simulink model "EXP1_EX13"  (R2021b)
settings: Solver=VariableStepAuto  StartTime=0.0  StopTime=20.0  RelTol=1e-3
values from neighbouring files (symbols this model uses):
  kp = eye(2)    [EXP1.m]
  u1 = 0    [EXP1.m]
  u2 = 1    [EXP1.m]
settings Model: Creator=luang  LastModifiedBy=luang

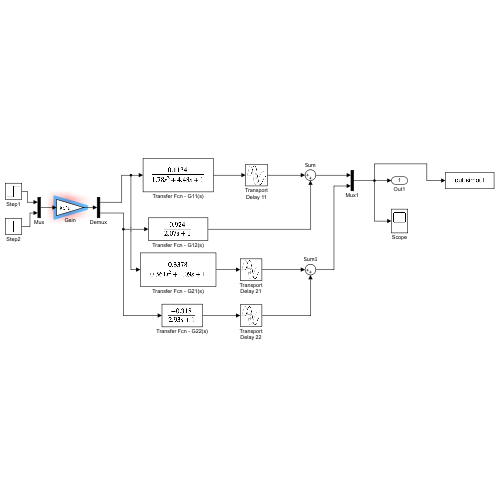
[thumbnail: Simulink's stored preview of the top-level diagram]
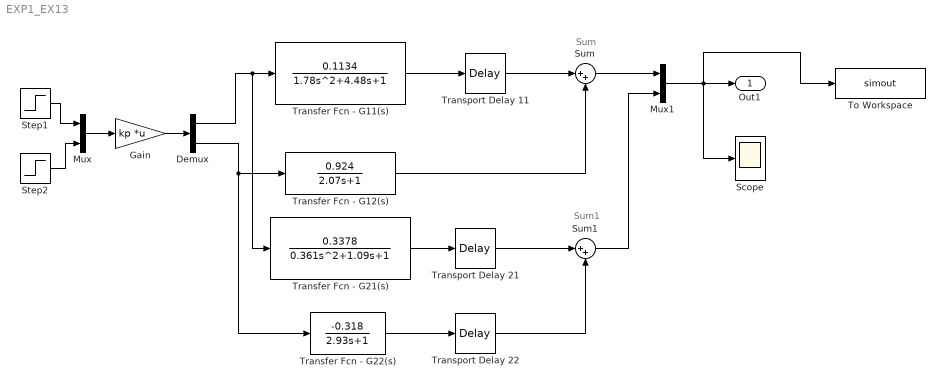
== system EXP1_EX13 ==
  note: Sum
  note: Sum1
  Demux : Demux  Outputs=2
  Gain : Gain  Gain=kp  Multiplication=Matrix(K*u)
  Mux : Mux  Inputs=2
  Mux1 : Mux  Inputs=2
  Scope : Scope
  Step1 : Step  After=u1  SampleTime=0
  Step2 : Step  After=u2  SampleTime=0
  Sum : Sum  Inputs=|++
  Sum1 : Sum  Inputs=|++
  To Workspace : ToWorkspace  VariableName=simout  SaveFormat=Structure With Time  SampleTime=-1
  Transfer Fcn - G11(s) : TransferFcn  Numerator=[0.1134]  Denominator=[1.78 4.48 1]  ContinuousStateAttributes='G11'
  Transfer Fcn - G12(s) : TransferFcn  Numerator=[0.924]  Denominator=[2.07 1]
  Transfer Fcn - G21(s) : TransferFcn  Numerator=[0.3378]  Denominator=[0.361 1.09 1]
  Transfer Fcn - G22(s) : TransferFcn  Numerator=[-0.318]  Denominator=[2.93 1]
  Transport Delay 11 : TransportDelay  DelayTime=0.72
  Transport Delay 21 : TransportDelay  DelayTime=0.3
  Transport Delay 22 : TransportDelay  DelayTime=1.29
  Out1 : Outport
  wires:
  Demux/2 -> Transfer Fcn - G12(s)/1, Transfer Fcn - G22(s)/1
  Transfer Fcn - G21(s)/1 -> Transport Delay 21/1
  Sum1/1 -> Mux1/2
  Mux1/1 -> To Workspace/1, Scope/1, Out1/1
  Demux/1 -> Transfer Fcn - G21(s)/1, Transfer Fcn - G11(s)/1
  Mux/1 -> Gain/1
  Step2/1 -> Mux/2
  Transport Delay 22/1 -> Sum1/2
  Sum/1 -> Mux1/1
  Transfer Fcn - G22(s)/1 -> Transport Delay 22/1
  Transport Delay 21/1 -> Sum1/1
  Transfer Fcn - G12(s)/1 -> Sum/2
  Gain/1 -> Demux/1
  Transfer Fcn - G11(s)/1 -> Transport Delay 11/1
  Transport Delay 11/1 -> Sum/1
  Step1/1 -> Mux/1
